simulink model "inductance"  (R2024a)
settings: Solver=VariableStepAuto  StartTime=0.0  StopTime=10.0  RelTol=1e-3
undefined symbols (not defined in the file): a, L0, Ld
settings Model: Creator=Bocchio  LastModifiedBy=Bocchio

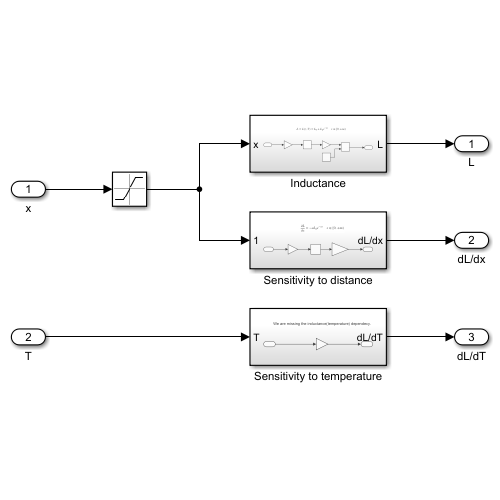
[thumbnail: Simulink's stored preview of the top-level diagram]
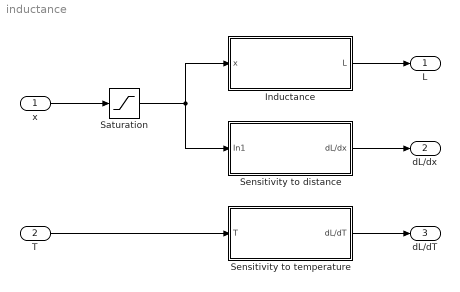
== system inductance ==
  x : Inport
  T : Inport  Port=2
  Inductance : Subsystem
  Saturation : Saturate  UpperLimit=+inf  LowerLimit=0
  Sensitivity to distance : Subsystem
  Sensitivity to temperature : Subsystem
  L : Outport
  dL/dx : Outport  Port=2
  dL/dT : Outport  Port=3
  wires:
  T/1 -> Sensitivity to temperature/1(T)
  x/1 -> Saturation/1
  Sensitivity to distance/1(dL/dx) -> dL/dx/1
  Sensitivity to temperature/1(dL/dT) -> dL/dT/1
  Saturation/1 -> Inductance/1(x), Sensitivity to distance/1(In1)
  Inductance/1(L) -> L/1

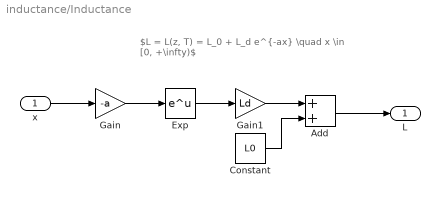
== system inductance/Inductance ==
  note: $L = L(z, T) = L_0 + L_d e^{-ax} \quad x \in [0, +\infty)$
  x : Inport
  Add : Sum
  Constant : Constant  Value=L0
  Exp : Math
  Gain : Gain  Gain=-a
  Gain1 : Gain  Gain=Ld
  L : Outport
  wires:
  x/1 -> Gain/1
  Gain1/1 -> Add/1
  Add/1 -> L/1
  Constant/1 -> Add/2
  Gain/1 -> Exp/1
  Exp/1 -> Gain1/1

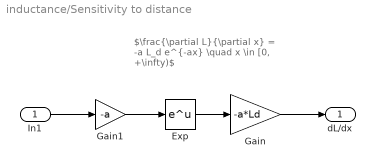
== system inductance/Sensitivity to distance ==
  note: $\frac{\partial L}{\partial x} = -a L_d e^{-ax} \quad x \in [0, +\infty)$
  In1 : Inport
  Exp : Math
  Gain : Gain  Gain=-a*Ld
  Gain1 : Gain  Gain=-a
  dL/dx : Outport
  wires:
  Gain1/1 -> Exp/1
  Gain/1 -> dL/dx/1
  Exp/1 -> Gain/1
  In1/1 -> Gain1/1

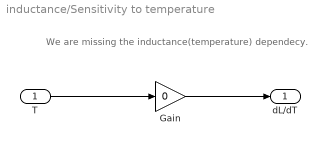
== system inductance/Sensitivity to temperature ==
  note: We are missing the inductance(temperature) dependecy.
  T : Inport
  Gain : Gain  Gain=0
  dL/dT : Outport
  wires:
  T/1 -> Gain/1
  Gain/1 -> dL/dT/1
